simulink model "sar_simulink"  (R2024a)
settings: Solver=FixedStepAuto  StartTime=0.0  StopTime=N/fs  RelTol=1e-3
values from neighbouring files (symbols this model uses):
  fss = 75e6    (= 75000000)    [A_read_data.m]
  R = 1/3    (= 0.333333333333)    [A_read_data.m]
  Rs = 37.5e6    (= 37500000)    [A_read_data.m]
  Ts = 1/fs    (= 2e-08)    [A_read_data.m]
libraries: commsync2 x2, dspfdesign x1, commrflib2 x1, commfilt2 x1, dspsigops x1
settings Model: Creator=Anthony  LastModifiedBy=25379
settings SolverCC: MinimalZcImpactIntegration=on
settings OptimizationCC: SimCompilerOptimization=on
settings DebuggingCC: ReadBeforeWriteMsg=DisableAll  WriteAfterWriteMsg=DisableAll  WriteAfterReadMsg=DisableAll  MultiTaskDSMMsg=none
settings ModelReferenceCC: UpdateModelReferenceTargets=IfOutOfDate  EnableRefExpFcnMdlSchedulingChecks=on
settings SFSimCC: SFSimEcho=off  SimHardwareAcceleration=native  SimTargetLang=C++  GPUAcceleration=on  SimDLTargetLibrary=cudnn
settings RTWCC: GPUComputeCapability=3.5

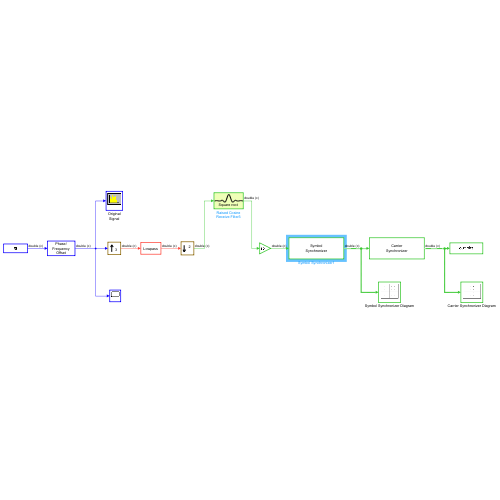
[thumbnail: Simulink's stored preview of the top-level diagram]
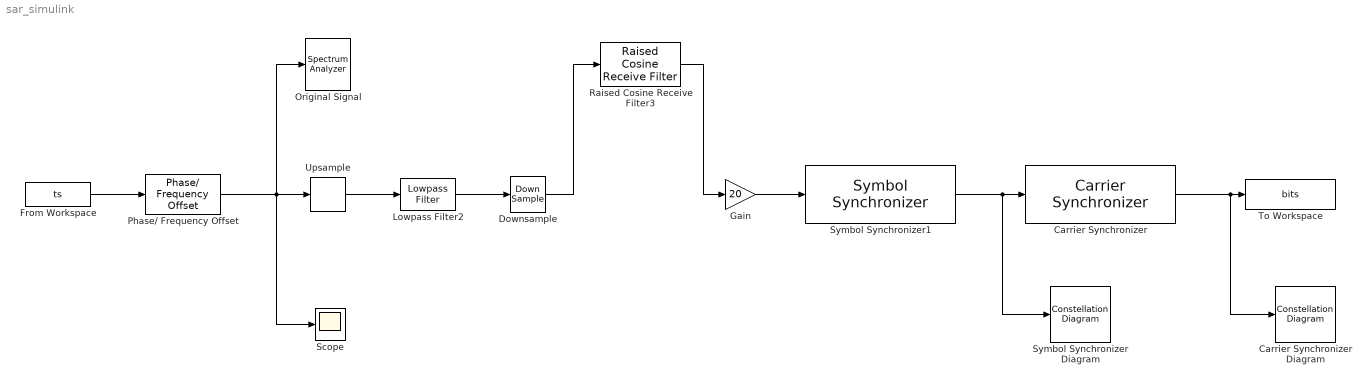
== system sar_simulink ==
  Carrier Synchronizer : commsync2/Carrier Synchronizer  Modulation=QPSK  ModulationPhaseOffset=Auto  CustomPhaseOffset=0  SamplesPerSymbol=fss/Rs  DampingFactor=10  NormalizedLoopBandwidth=0.35  EstimatedPhaseErrorOutputPort=off  SimulateUsing=Code generation
  Carrier Synchronizer Diagram : ConstellationDiagram  WindowPosition=[1037.000000,347.000000,519.000000,494.000000,]  Visible=on  ScopeFrameLocation=window  SamplesPerSymbol=fss/Rs  SymbolsToDisplaySource=Property  SymbolsToDisplay=1000  XLimits=[-1.69,1.69]  YLimits=[-1.48,1.48]
  Downsample : DownSample  RateOptions=Allow multirate processing  AllowArbitraryFixedInput=on
  From Workspace : FromWorkspace  VariableName=ts  SampleTime=Ts  Interpolate=off  OutputAfterFinalValue=Setting to zero
  Gain : Gain  Gain=20
  Lowpass Filter2 : dspfdesign/Lowpass Filter  FilterType=FIR  DesignForMinimumOrder=on  FilterOrder=50  PassbandFrequency=freqStart  StopbandFrequency=freqEnd  PassbandRipple=0.1  StopbandAttenuation=80  SampleRateMode=Specify on dialog  SampleRate=fss*6  SimulateUsing=Code generation  roundingMode=Floor  coeffsDataTypeStr=fixdt(1,16)
  Original Signal : SpectrumAnalyzer  WindowPosition=[374.000000,279.000000,958.000000,508.000000,]  Visible=on  ScopeFrameLocation=window  SampleRate=300000000  AxesScaling=Manual  AveragingMethod=Exponential  YLimits=[-58.27050501,-10.02185166]  AllowFFTLengthLessThanSamplesPerUpdate=on
  Phase/ Frequency Offset : commrflib2/Phase// Frequency Offset  phaseOffset=0  freqPort=off  freqOffset=0
  Raised Cosine Receive Filter3 : commfilt2/Raised Cosine Receive Filter  filtType=Square root  R=R  filtSpan=10  N=fss/Rs  downFactor=1  downOffset=0  filterGain=1  RateOptions=Allow multirate processing  framing=Allow multirate processing  checkCoeff=off  variableName=rcRxFilt3  currentFiltSpan=8  D=(8)/2  inputOffset=0  sampMode=Mute  saveAsFlag=0  rateMode=Downsampling  checkGain=Normalized  launchFVT=on  roundingMode=Floor  overflowMode=off  coeffDataTypeStr=Inherit: Same word length as input  coeffMin=[]  coeffMax=[]  coeffLastDataTypeStr=Inherit: Same word length as input  accumDataTypeStr=Inherit: Same as product output  accumLastDataTypeStr=Inherit: Same as product output  outputDataTypeStr=Inherit: Same as accumulator  outputMin=[]  outputMax=[]  outputLastDataTypeStr=Inherit: Same as accumulator
  Scope : Scope
  Symbol Synchronizer Diagram : ConstellationDiagram  WindowPosition=[333.000000,142.000000,518.000000,491.000000,]  Visible=on  ScopeFrameLocation=window  SamplesPerSymbol=fss/Rs  SymbolsToDisplaySource=Property  SymbolsToDisplay=1000  XLimits=[-1.69,1.69]  YLimits=[-1.48,1.48]
  Symbol Synchronizer1 : commsync2/Symbol Synchronizer  Modulation=PAM/PSK/QAM  TimingErrorDetector=Gardner (non-data-aided)  SamplesPerSymbol=fss/Rs  DampingFactor=10  NormalizedLoopBandwidth=0.001  DetectorGain=1  TimingErrorOutputPort=off  SimulateUsing=Code generation
  To Workspace : ToWorkspace  VariableName=bits  SaveFormat=Timeseries  SampleTime=-1
  Upsample : dspsigops/Upsample  FactorSource=Dialog parameter  N=3  Nmax=16  phase=0  RateOptions=Allow multirate processing  ic=0  mode=Unused parameter value
  wires:
  Phase/ Frequency Offset/1 -> Scope/1, Upsample/1, Original Signal/1
  Lowpass Filter2/1 -> Downsample/1
  Symbol Synchronizer1/1 -> Carrier Synchronizer/1, Symbol Synchronizer Diagram/1
  Carrier Synchronizer/1 -> To Workspace/1, Carrier Synchronizer Diagram/1
  Downsample/1 -> Raised Cosine Receive Filter3/1
  Upsample/1 -> Lowpass Filter2/1
  From Workspace/1 -> Phase/ Frequency Offset/1
  Gain/1 -> Symbol Synchronizer1/1
  Raised Cosine Receive Filter3/1 -> Gain/1
